simulink model "Project"  (R2020b)
settings: Solver=VariableStepAuto  StartTime=0.0  StopTime=100  RelTol=1e-3
undefined symbols (not defined in the file or in its folder): RES, SET, sigbuilder_block
settings Model: EnablePacing=on  PacingRate=2  Creator=99003729  LastModifiedBy=Admin

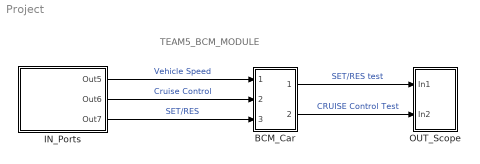
== system Project ==
  note: TEAM5_BCM_MODULE
  BCM_Car : Subsystem
  IN_Ports : Subsystem
  OUT_Scope : Subsystem
  wires:
  IN_Ports/1(Out5) -> BCM_Car/1(In1)  "Vehicle Speed"
  IN_Ports/3(Out7) -> BCM_Car/3(In3)  "SET/RES"
  IN_Ports/2(Out6) -> BCM_Car/2(In2)  "Cruise Control"
  BCM_Car/1(Out1) -> OUT_Scope/1(In1)  "SET/RES test"
  BCM_Car/2(Out2) -> OUT_Scope/2(In2)  "CRUISE Control Test"

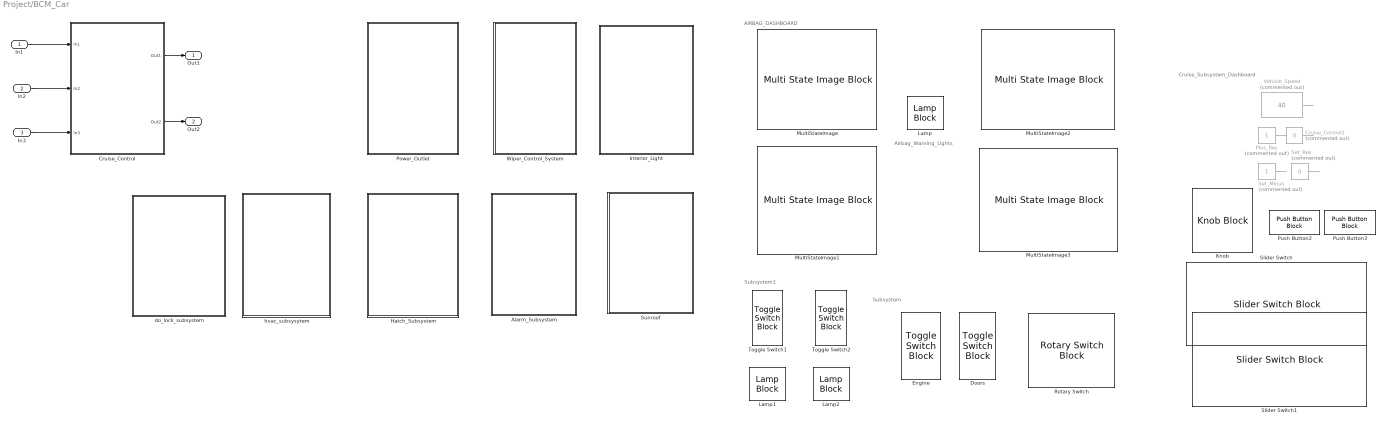
== system Project/BCM_Car ==
  note: AIRBAG_DASHBOARD
  note: Airbag_Warning_Lights
  note: Cruise_Subsystem_Dashboard
  note: Subsystem
  note: Subsystem1
  In1 : Inport
  In2 : Inport  Port=2
  In3 : Inport  Port=3
  Alarm_Subsystem : Subsystem
  Cruise_Control : Subsystem
  Cruise_Control1 : Constant  Commented=on  Value=0
  Doors : ToggleSwitchBlock
      settings: Values={{'Off', 'On'}, [0 1]}
  Engine : ToggleSwitchBlock
      settings: Values={{'Off', 'On'}, [0 1]}
  Hatch_Subsystem : Subsystem
  Interior_Light : Subsystem
  Knob : KnobBlock
  Lamp : LampBlock
  Lamp1 : LampBlock
  Lamp2 : LampBlock
  MultiStateImage{,1..3} (4 alike) : MultiStateImageBlock
  Plus_Res : Constant  Commented=on
  Power_Outlet : Subsystem
  Push Button2 : PushButtonBlock  ButtonText=SET-
  Push Button3 : PushButtonBlock  ButtonText=+RES
  Rotary Switch : RotarySwitchBlock
      settings: Values={{'Off', 'Button', 'Double Press'}, [0 1 2]}
  Set_Minus : Constant  Commented=on
  Set_Res : Constant  Commented=on  Value=0
  Slider Switch : SliderSwitchBlock
      settings: Values={{'Cruise Control Off', 'Cruise Control On'}, [0 1]}
  Slider Switch1 : SliderSwitchBlock
      settings: Values={{'Off with set speed', 'Resume set speed'}, [0 1]}
  Sunroof : Subsystem
  Toggle Switch1 : ToggleSwitchBlock
      settings: Values={{'Bonnet Off', 'Bonnet On'}, [0 1]}
  Toggle Switch2 : ToggleSwitchBlock
      settings: Values={{'Bonnet Off', 'Bonnet On'}, [0 1]}
  Vehicle_Speed : Constant  Commented=on  Value=40
  Wiper_Control_System : Subsystem
  do_lock_subsystem : Subsystem
  hvac_subsysytem : Subsystem
  Out1 : Outport
  Out2 : Outport  Port=2
  wires:
  Set_Res/1 -> ?
  Plus_Res/1 -> ?
  Vehicle_Speed/1 -> ?
  Set_Minus/1 -> ?
  Cruise_Control1/1 -> ?
  In1/1 -> Cruise_Control/1(In1)
  In2/1 -> Cruise_Control/2(In2)
  In3/1 -> Cruise_Control/3(In3)
  Cruise_Control/1(Out1) -> Out1/1
  Cruise_Control/2(Out2) -> Out2/1

== system Project/IN_Ports ==
  note: Airbag_And_Cruise_InPorts
  Alarm_and_Hatch_InPorts : Subsystem
  Hvac_and_Door_InPorts : Subsystem
  Square_Signals : Subsystem  Tag=STV Subsys  LoadFcn=sigbuilder_block('load');  StartFcn=sigbuilder_block('start');  StopFcn=sigbuilder_block('stop');  ClipboardFcn=sigbuilder_block('clipboard');  mask(Sigbuilder block){tuvar=[0:10]}
      mask help: Simulink:masks:SigbuilderBlock_MD
      mask init:
      | if ~strcmp(get_param(bdroot(gcbh),'SimulationStatus'),'stopped') tuvar = sigbuilder_block('maskInit'); end
      settings: CopyFcn=sigbuilder_block('copy');  DeleteFcn=sigbuilder_block('delete');  ModelCloseFcn=sigbuilder_block('modelClose');  PreSaveFcn=sigbuilder_block('preSave');  PauseFcn=sigbuilder_block('pause');  ContinueFcn=sigbuilder_block('continue');  NameChangeFcn=sigbuilder_block('namechange');  OpenFcn=sigbuilder_block('open',[6 30 1012.5 447.75 ]);  CloseFcn=sigbuilder_block('close');
      mask Display: plot(0, 0, 100, 100,[2, 2, 32, 32, 2], [68, 8, 8, 68, 68],[32, 2], [38, 38], [32, 19, 2],[53, 60, 44], [32, 17, 17, 2],[16, 16, 31, 31]);txt = getActiveGroup(gcbh);text(2, 100, txt,'verticalAlignment', 'top');
  Sunroof_and_InteriorLights_InPorts : Subsystem
  Wiper_and_Power_InPorts : Subsystem
  Out5 : Outport
  Out6 : Outport  Port=2
  Out7 : Outport  Port=3
  wires:
  Square_Signals/2(Cruise_Control) -> Out6/1  "Cruise_Control"
  Square_Signals/1(Vehicle_Speed) -> Out5/1  "Vehicle_Spped"
  Square_Signals/3(Set_Res_Control) -> Out7/1  "Set_Res_Control"

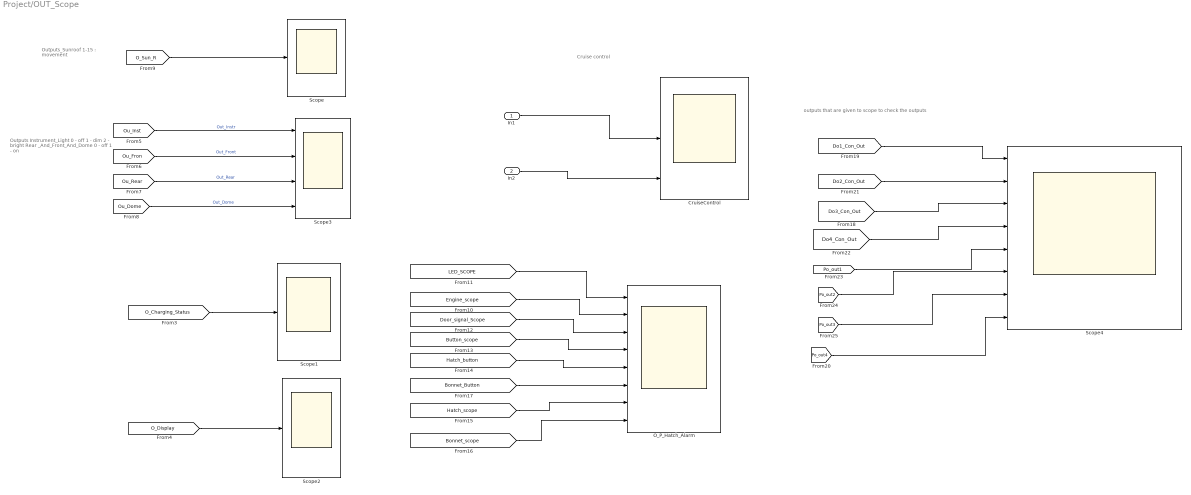
== system Project/OUT_Scope ==
  note: Cruise control
  note: Outputs
      | Instrument_Light
      | 0 - off
      | 1 - dim
      | 2 - bright
      | Rear _And_Front_And_Dome
      | 0 - off
      | 1 - on
  note: Outputs_Sunroof
      | 1-15 : movement
  note: outputs that are given to scope to check the outputs
  In1 : Inport
  In2 : Inport  Port=2
  CruiseControl : Scope  NumInputPorts=3
  O_P_Hatch_Alarm : Scope  NumInputPorts=8
  Scope : Scope
  Scope1 : Scope
  Scope2 : Scope
  Scope3 : Scope  NumInputPorts=4
  Scope4 : Scope  NumInputPorts=8
  wires:
  [O_Charging_Status] -> Scope1/1
  [O_Display] -> Scope2/1
  [Ou_Inst] -> Scope3/1  "Out_Instr"
  [Ou_Fron] -> Scope3/2  "Out_Front"
  [Ou_Rear] -> Scope3/3  "Out_Rear"
  [Ou_Dome] -> Scope3/4  "Out_Dome"
  [O_Sun_R] -> Scope/1
  [Bonnet_Button] -> O_P_Hatch_Alarm/6
  [Bonnet_scope] -> O_P_Hatch_Alarm/8
  [Door_signal_Scope] -> O_P_Hatch_Alarm/3
  [Hatch_button] -> O_P_Hatch_Alarm/5
  [Hatch_scope] -> O_P_Hatch_Alarm/7
  [LED_SCOPE] -> O_P_Hatch_Alarm/1
  [Engine_scope] -> O_P_Hatch_Alarm/2
  [Button_scope] -> O_P_Hatch_Alarm/4
  [Po_out3] -> Scope4/7
  [Po_out4] -> Scope4/8
  [Do3_Con_Out] -> Scope4/3
  [Po_out1] -> Scope4/5
  [Do1_Con_Out] -> Scope4/1
  [Do4_Con_Out] -> Scope4/4
  [Po_out2] -> Scope4/6
  [Do2_Con_Out] -> Scope4/2
  In1/1 -> CruiseControl/2
  In2/1 -> CruiseControl/3

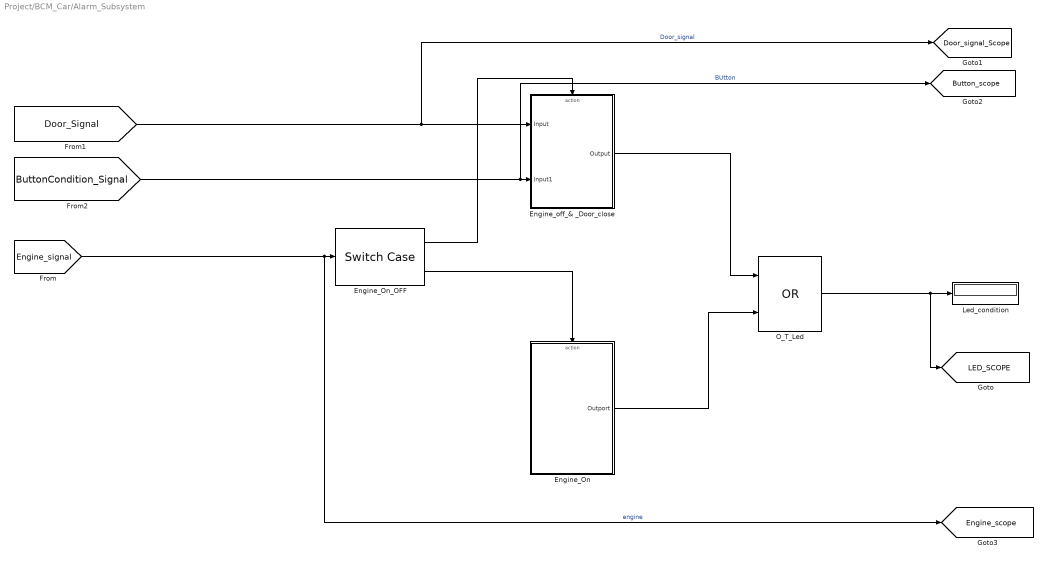
== system Project/BCM_Car/Alarm_Subsystem ==
  Engine_On : Subsystem  TreatAsAtomicUnit=on
  Engine_On_OFF : SwitchCase  CaseConditions={0,1}  ShowDefaultCase=off
  Engine_off_& _Door_close : Subsystem  TreatAsAtomicUnit=on
  Led_condition : Display
  O_T_Led : Logic  Operator=OR  IconShape=distinctive  AllPortsSameDT=off  OutDataTypeStr=boolean
  tag scope: Button_scope=global, Door_signal_Scope=global, Engine_scope=global, LED_SCOPE=global
  wires:
  O_T_Led/1 -> [LED_SCOPE], Led_condition/1
  Engine_On_OFF/1 -> Engine_off_& _Door_close/Action
  Engine_On_OFF/2 -> Engine_On/Action
  Engine_On/1(Outport) -> O_T_Led/2
  Engine_off_& _Door_close/1(Output) -> O_T_Led/1
  [Engine_signal] -> [Engine_scope], Engine_On_OFF/1  "engine"
  [Door_Signal] -> [Door_signal_Scope], Engine_off_& _Door_close/1(Input)  "Door_signal"
  [ButtonCondition_Signal] -> [Button_scope], Engine_off_& _Door_close/2(Input1)  "BUtton"

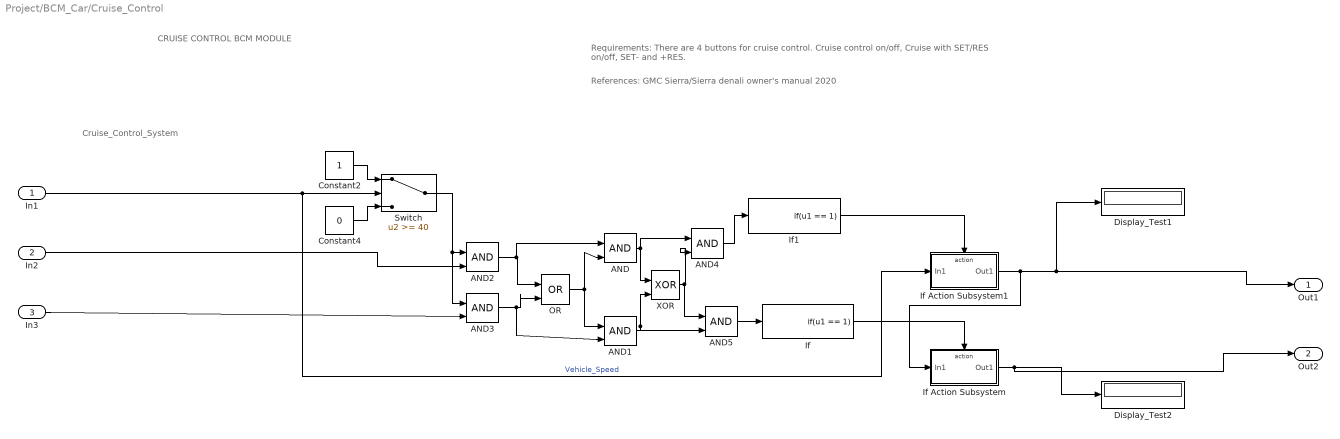
== system Project/BCM_Car/Cruise_Control ==
  note: Cruise_Control_System
  note: CRUISE CONTROL BCM MODULE
  note: References: GMC Sierra/Sierra denali owner's manual 2020
  note: Requirements: There are 4 buttons for cruise control. Cruise control on/off, Cruise with SET/RES on/off, SET- and +RES.
  In1 : Inport
  In2 : Inport  Port=2
  In3 : Inport  Port=3
  AND{,1..5} (6 alike) : Logic  IconShape=distinctive  AllPortsSameDT=off  OutDataTypeStr=boolean
  Constant2 : Constant
  Constant4 : Constant  Value=0
  Display_Test1 : Display
  Display_Test2 : Display
  If : If  IfExpression=u1 == 1  ShowElse=off
  If Action Subsystem : Subsystem  TreatAsAtomicUnit=on
  If Action Subsystem1 : Subsystem  TreatAsAtomicUnit=on
  If1 : If  IfExpression=u1 == 1  ShowElse=off
  OR : Logic  Operator=OR  IconShape=distinctive  AllPortsSameDT=off  OutDataTypeStr=boolean
  Switch : Switch  Threshold=40
  XOR : Logic  Operator=XOR  IconShape=distinctive  AllPortsSameDT=off  OutDataTypeStr=boolean
  Out1 : Outport
  Out2 : Outport  Port=2
  wires:
  In3/1 -> AND3/2
  AND5/1 -> If/1
  If1/1 -> If Action Subsystem1/Action
  If/1 -> If Action Subsystem/Action
  If Action Subsystem/1(Out1) -> Out2/1, Display_Test2/1
  AND/1 -> AND4/1, XOR/1
  XOR/1 -> AND5/1, AND4/2
  In1/1 -> If Action Subsystem1/1(In1), Switch/2  "Vehicle_Speed"
  OR/1 -> AND1/1, AND/2
  AND2/1 -> AND/1, OR/1
  In2/1 -> AND2/2
  Constant4/1 -> Switch/3
  AND3/1 -> AND1/2, OR/2
  AND1/1 -> XOR/2, AND5/2
  Switch/1 -> AND3/1, AND2/1
  Constant2/1 -> Switch/1
  AND4/1 -> If1/1
  If Action Subsystem1/1(Out1) -> If Action Subsystem/1(In1), Out1/1, Display_Test1/1

== system Project/BCM_Car/Hatch_Subsystem ==
  H_B_condition : Stateflow chart  TreatAsAtomicUnit=on
  Hatch_Bonnet_condition : Display
  OR : Logic  Operator=OR  IconShape=distinctive  AllPortsSameDT=off  OutDataTypeStr=boolean
  tag scope: Bonnet_scope=global, Hatch_scope=global
  wires:
  [Bonnet_Button] -> H_B_condition/1(BonnetButton)
  OR/1 -> Hatch_Bonnet_condition/1
  H_B_condition/1(y) -> [Bonnet_scope], OR/1
  H_B_condition/2(x) -> [Hatch_scope], OR/2
  [Hatch_button] -> H_B_condition/2(hatchButton)

== system Project/BCM_Car/Interior_Light ==
  Function_Light : MATLAB Function  TreatAsAtomicUnit=on
  tag scope: Ou_Dome=global, Ou_Fron=global, Ou_Inst=global, Ou_Rear=global
  wires:
  [Dome_L] -> Function_Light/4(u3)
  [Inst_Light] -> Function_Light/1(u)
  [Fron_Read_Light] -> Function_Light/2(u1)
  [Rear_Read_Light] -> Function_Light/3(u2)
  Function_Light/1(y) -> [Ou_Inst]
  Function_Light/2(y1) -> [Ou_Fron]
  Function_Light/3(y2) -> [Ou_Rear]
  Function_Light/4(y3) -> [Ou_Dome]

== system Project/BCM_Car/Power_Outlet ==
  note: Inputs_Engine
      |
      | 0: Engine is Off
      | 1: Engine is On
  I_Const_0 : Constant  Value=0
  I_Const_1 : Constant
  Power_Outlet_Subsystem : Subsystem
  Switch : Switch  Criteria=u2 > Threshold
  wires:
  I_Const_0/1 -> Switch/3
  [Engine_Input] -> Switch/2
  Switch/1 -> Power_Outlet_Subsystem/1(In1)
  I_Const_1/1 -> Switch/1

== system Project/BCM_Car/Sunroof ==
  Function_Sun : MATLAB Function  TreatAsAtomicUnit=on
  tag scope: O_Sun_R=global
  wires:
  Function_Sun/1(y) -> [O_Sun_R]  "Out_Sun"
  [I_Sensor] -> Function_Sun/2(v)
  [In_Su_Roof] -> Function_Sun/1(u)

== system Project/BCM_Car/Wiper_Control_System ==
  note: 1:Wiper is in Low Speed
      | 2:Wiper is in Medium Speed
      | 3:Wiper is in High Speed
      | 4:Wiper is in Mist
      | 5:Wiper is in OFF
  High_Speed : Constant  Value=3
  Low_Speed : Constant
  Medium_Speed : Constant  Value=2
  Mist : Constant  Value=4
  Multiport Switch for input conditions : MultiPortSwitch  Inputs=5  DiagnosticForDefault=None
  Off : Constant  Value=5
  tag scope: O_Display=global
  wires:
  [In_Value_Wiper] -> Multiport Switch for input conditions/1
  Low_Speed/1 -> Multiport Switch for input conditions/2
  Mist/1 -> Multiport Switch for input conditions/5
  Medium_Speed/1 -> Multiport Switch for input conditions/3
  Multiport Switch for input conditions/1 -> [O_Display]
  High_Speed/1 -> Multiport Switch for input conditions/4
  Off/1 -> Multiport Switch for input conditions/6

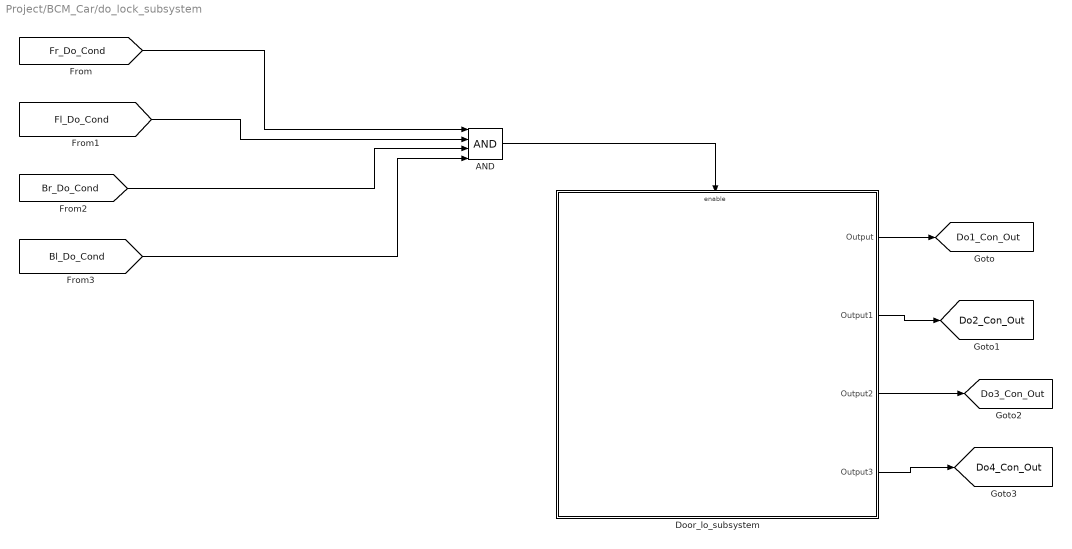
== system Project/BCM_Car/do_lock_subsystem ==
  AND : Logic  Inputs=4  IconShape=distinctive  AllPortsSameDT=off  OutDataTypeStr=boolean
  Door_lo_subsystem : Subsystem  TreatAsAtomicUnit=on
  tag scope: Do1_Con_Out=global, Do2_Con_Out=global, Do3_Con_Out=global, Do4_Con_Out=global
  wires:
  [Br_Do_Cond] -> AND/3
  [Fl_Do_Cond] -> AND/2
  [Fr_Do_Cond] -> AND/1
  AND/1 -> Door_lo_subsystem/Enable
  [Bl_Do_Cond] -> AND/4
  Door_lo_subsystem/1(Output) -> [Do1_Con_Out]
  Door_lo_subsystem/2(Output1) -> [Do2_Con_Out]
  Door_lo_subsystem/3(Output2) -> [Do3_Con_Out]
  Door_lo_subsystem/4(Output3) -> [Do4_Con_Out]

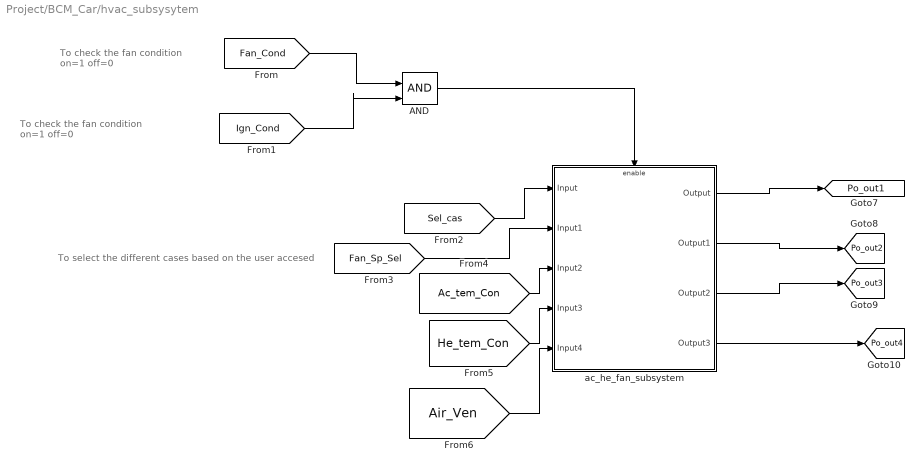
== system Project/BCM_Car/hvac_subsysytem ==
  note: To select the different cases based on the user accesed
  note: To check the fan condition
      | on=1
      | off=0
  note: To check the fan condition
      | on=1
      | off=0
  AND : Logic  IconShape=distinctive  AllPortsSameDT=off  OutDataTypeStr=boolean
  ac_he_fan_subsystem : Subsystem
  tag scope: Po_out1=global, Po_out2=global, Po_out3=global, Po_out4=global
  wires:
  [Fan_Cond] -> AND/1
  [Ign_Cond] -> AND/2
  AND/1 -> ac_he_fan_subsystem/Enable
  [Sel_cas] -> ac_he_fan_subsystem/1(Input)
  [Fan_Sp_Sel] -> ac_he_fan_subsystem/2(Input1)
  [Ac_tem_Con] -> ac_he_fan_subsystem/3(Input2)
  [He_tem_Con] -> ac_he_fan_subsystem/4(Input3)
  ac_he_fan_subsystem/1(Output) -> [Po_out1]
  ac_he_fan_subsystem/2(Output1) -> [Po_out2]
  ac_he_fan_subsystem/3(Output2) -> [Po_out3]
  ac_he_fan_subsystem/4(Output3) -> [Po_out4]
  [Air_Ven] -> ac_he_fan_subsystem/5(Input4)

== system Project/IN_Ports/Alarm_and_Hatch_InPorts ==
  Signal Builder : Subsystem  Tag=STV Subsys  LoadFcn=sigbuilder_block('load');  StartFcn=sigbuilder_block('start');  StopFcn=sigbuilder_block('stop');  ClipboardFcn=sigbuilder_block('clipboard');  mask(Sigbuilder block){tuvar=[0:10]}
      mask help: Simulink:masks:SigbuilderBlock_MD
      mask init:
      | if ~strcmp(get_param(bdroot(gcbh),'SimulationStatus'),'stopped') tuvar = sigbuilder_block('maskInit'); end
      settings: CopyFcn=sigbuilder_block('copy');  DeleteFcn=sigbuilder_block('delete');  ModelCloseFcn=sigbuilder_block('modelClose');  PreSaveFcn=sigbuilder_block('preSave');  PauseFcn=sigbuilder_block('pause');  ContinueFcn=sigbuilder_block('continue');  NameChangeFcn=sigbuilder_block('namechange');  OpenFcn=sigbuilder_block('open',[437.6 199.2 550.4 400 ]);  CloseFcn=sigbuilder_block('close');
      mask Display: plot(0, 0, 100, 100,[2, 2, 32, 32, 2], [68, 8, 8, 68, 68],[32, 2], [38, 38], [32, 19, 2],[53, 60, 44], [32, 17, 17, 2],[16, 16, 31, 31]);txt = getActiveGroup(gcbh);text(2, 100, txt,'verticalAlignment', 'top');
  tag scope: Bonnet_Button=global, ButtonCondition_Signal=global, Door_Signal=global, Engine_signal=global, Hatch_button=global
  wires:
  Signal Builder/1(Engine_Signal) -> [Engine_signal]
  Signal Builder/5(Hatch_button) -> [Hatch_button]
  Signal Builder/4(Bonnet_button) -> [Bonnet_Button]
  Signal Builder/2(Door_signal) -> [Door_Signal]
  Signal Builder/3(ButtonCondition_Signal) -> [ButtonCondition_Signal]

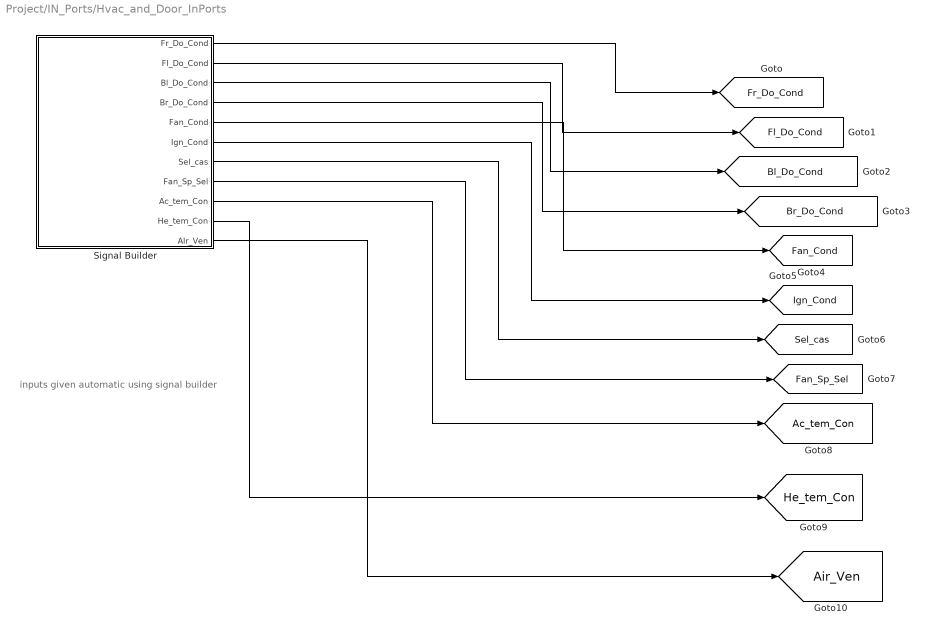
== system Project/IN_Ports/Hvac_and_Door_InPorts ==
  note: inputs given automatic using signal builder
  Signal Builder : Subsystem  Tag=STV Subsys  LoadFcn=sigbuilder_block('load');  StartFcn=sigbuilder_block('start');  StopFcn=sigbuilder_block('stop');  ClipboardFcn=sigbuilder_block('clipboard');  mask(Sigbuilder block){tuvar=[0:10]}
      mask help: Simulink:masks:SigbuilderBlock_MD
      mask init:
      | if ~strcmp(get_param(bdroot(gcbh),'SimulationStatus'),'stopped') tuvar = sigbuilder_block('maskInit'); end
      settings: CopyFcn=sigbuilder_block('copy');  DeleteFcn=sigbuilder_block('delete');  ModelCloseFcn=sigbuilder_block('modelClose');  PreSaveFcn=sigbuilder_block('preSave');  PauseFcn=sigbuilder_block('pause');  ContinueFcn=sigbuilder_block('continue');  NameChangeFcn=sigbuilder_block('namechange');  OpenFcn=sigbuilder_block('open',[544.5 115.5 550.5 399.75 ]);  CloseFcn=sigbuilder_block('close');
      mask Display: plot(0, 0, 100, 100,[2, 2, 32, 32, 2], [68, 8, 8, 68, 68],[32, 2], [38, 38], [32, 19, 2],[53, 60, 44], [32, 17, 17, 2],[16, 16, 31, 31]);txt = getActiveGroup(gcbh);text(2, 100, txt,'verticalAlignment', 'top');
  tag scope: Ac_tem_Con=global, Air_Ven=global, Bl_Do_Cond=global, Br_Do_Cond=global, Fan_Cond=global, Fan_Sp_Sel=global, Fl_Do_Cond=global, Fr_Do_Cond=global, He_tem_Con=global, Ign_Cond=global, Sel_cas=global
  wires:
  Signal Builder/4(Br_Do_Cond) -> [Br_Do_Cond]
  Signal Builder/2(Fl_Do_Cond) -> [Fl_Do_Cond]
  Signal Builder/6(Ign_Cond) -> [Ign_Cond]
  Signal Builder/3(Bl_Do_Cond) -> [Bl_Do_Cond]
  Signal Builder/7(Sel_cas) -> [Sel_cas]
  Signal Builder/8(Fan_Sp_Sel) -> [Fan_Sp_Sel]
  Signal Builder/1(Fr_Do_Cond) -> [Fr_Do_Cond]
  Signal Builder/5(Fan_Cond) -> [Fan_Cond]
  Signal Builder/9(Ac_tem_Con) -> [Ac_tem_Con]
  Signal Builder/11(AIr_Ven) -> [Air_Ven]
  Signal Builder/10(He_tem_Con) -> [He_tem_Con]

== system Project/IN_Ports/Square_Signals ==
  Demux : Demux  Tag=STV Demux  Outputs=3
      settings: DisplayOption=none
  FromWs : FromWorkspace  Tag=STV FromWs  VariableName=tuvar
      SigBuilderData=|
      | common.afterFinalStr = 'Extrapolate'
      | common.sampleTime = 0
      | dataSet.timeRange = [0 100]
      | dataSet.name = 'Group 1'
      | sbobj.Groups.Name = 'Group 1'
      | sbobj.Groups.Signals(1).Name = 'Vehicle_Speed'
      | sbobj.Groups.Signals(1).XData = [0 5 10 15 20 25 30 35 40 45 50 55 60 65 70 75 80 85 90 95 100]
      | sbobj.Groups.Signals(1).YData = [50 50 50 50 50 50 50 50 50 50 50 50 50 50 50 50 50 50 50 50 50]
      | sbobj.Groups.Signals(2).Name = 'Cruise_Control'
      | sbobj.Groups.Signals(2).XData = [0 5 5 10 15 20 25 30 35 40 45 50 55 60 65 70 75 80 85 90 95 100]
      | sbobj.Groups.Signals(2).YData = [0 0 1 1 1 1 1 0 0 0 0 0 0 0 0 0 0 0 0 0 0 0]
      | sbobj.Groups.Signals(3).Name = 'Set_Res_Control'
      | sbobj.Groups.Signals(3).XData = [0 5 10 15 20 25 30 30 35 35 40 45 50 55 60 65 70 75 80 85 90 95 100]
      | sbobj.Groups.Signals(3).YData = [0 0 0 0 0 0 0 1 1 0 0 0 0 0 0 0 0 0 0 0 0 0 0]
      | sbobj.Groups.TimeRange = [0 100]
  Vehicle_Speed : Outport  Tag=STV Outport
  Cruise_Control : Outport  Tag=STV Outport  Port=2
  Set_Res_Control : Outport  Tag=STV Outport  Port=3
  wires:
  FromWs/1 -> Demux/1
  Demux/1 -> Vehicle_Speed/1
  Demux/2 -> Cruise_Control/1
  Demux/3 -> Set_Res_Control/1

== system Project/IN_Ports/Sunroof_and_InteriorLights_InPorts ==
  note: Inputs
      | Intrument_Light
      | 0 - off
      | 1 - dim
      | 2- bright
      | Front_And_Rear_Light
      | 0 - off
      | 1 - on
      | Dome_Light
      | 0 - off
      | 1 - on
  note: Sunroof_Inputs
      | 0 - off
      | 1 - siglepress
      | 2 - fullpress
      | Sensor_For_Object
      | 0 - no object
      | 1 - object
  Signal Builder2 : Subsystem  Tag=STV Subsys  LoadFcn=sigbuilder_block('load');  StartFcn=sigbuilder_block('start');  StopFcn=sigbuilder_block('stop');  ClipboardFcn=sigbuilder_block('clipboard');  mask(Sigbuilder block){tuvar=[0:10]}
      mask help: Simulink:masks:SigbuilderBlock_MD
      mask init:
      | if ~strcmp(get_param(bdroot(gcbh),'SimulationStatus'),'stopped') tuvar = sigbuilder_block('maskInit'); end
      settings: CopyFcn=sigbuilder_block('copy');  DeleteFcn=sigbuilder_block('delete');  ModelCloseFcn=sigbuilder_block('modelClose');  PreSaveFcn=sigbuilder_block('preSave');  PauseFcn=sigbuilder_block('pause');  ContinueFcn=sigbuilder_block('continue');  NameChangeFcn=sigbuilder_block('namechange');  OpenFcn=sigbuilder_block('open',[373.5 207 544.5 355.5 ]);  CloseFcn=sigbuilder_block('close');
      mask Display: plot(0, 0, 100, 100,[2, 2, 32, 32, 2], [68, 8, 8, 68, 68],[32, 2], [38, 38], [32, 19, 2],[53, 60, 44], [32, 17, 17, 2],[16, 16, 31, 31]);txt = getActiveGroup(gcbh);text(2, 100, txt,'verticalAlignment', 'top');
  Signal Builder3 : Subsystem  Tag=STV Subsys  LoadFcn=sigbuilder_block('load');  StartFcn=sigbuilder_block('start');  StopFcn=sigbuilder_block('stop');  ClipboardFcn=sigbuilder_block('clipboard');  mask(Sigbuilder block){tuvar=[0:10]}
      mask help: Simulink:masks:SigbuilderBlock_MD
      mask init:
      | if ~strcmp(get_param(bdroot(gcbh),'SimulationStatus'),'stopped') tuvar = sigbuilder_block('maskInit'); end
      settings: CopyFcn=sigbuilder_block('copy');  DeleteFcn=sigbuilder_block('delete');  ModelCloseFcn=sigbuilder_block('modelClose');  PreSaveFcn=sigbuilder_block('preSave');  PauseFcn=sigbuilder_block('pause');  ContinueFcn=sigbuilder_block('continue');  NameChangeFcn=sigbuilder_block('namechange');  OpenFcn=sigbuilder_block('open',[591 352.5 550.5 359.25 ]);  CloseFcn=sigbuilder_block('close');
      mask Display: plot(0, 0, 100, 100,[2, 2, 32, 32, 2], [68, 8, 8, 68, 68],[32, 2], [38, 38], [32, 19, 2],[53, 60, 44], [32, 17, 17, 2],[16, 16, 31, 31]);txt = getActiveGroup(gcbh);text(2, 100, txt,'verticalAlignment', 'top');
  tag scope: Dome_L=global, Fron_Read_Light=global, I_Sensor=global, In_Su_Roof=global, Inst_Light=global, Rear_Read_Light=global
  wires:
  Signal Builder2/1(Fron_Read_Light) -> [Fron_Read_Light]
  Signal Builder3/2(I_Sensor) -> [I_Sensor]
  Signal Builder2/3(Dome_L) -> [Dome_L]
  Signal Builder2/2(Rear_Read_Light) -> [Rear_Read_Light]
  Signal Builder3/1(In_Su_Roof) -> [In_Su_Roof]
  Signal Builder2/4(Inst_Light) -> [Inst_Light]

== system Project/IN_Ports/Wiper_and_Power_InPorts ==
  note: Inputs_Engine
      |
      | 0: Engine is Off
      | 1: Engine is On
  note: Input_Wiper_Control
      | 1:Low Speed
      | 2:Medium Speed
      | 3:High Speed
      | 4:Mist
      | 5:Off
  Signal Builder : Subsystem  Tag=STV Subsys  LoadFcn=sigbuilder_block('load');  StartFcn=sigbuilder_block('start');  StopFcn=sigbuilder_block('stop');  ClipboardFcn=sigbuilder_block('clipboard');  mask(Sigbuilder block){tuvar=[0:10]}
      mask help: Simulink:masks:SigbuilderBlock_MD
      mask init:
      | if ~strcmp(get_param(bdroot(gcbh),'SimulationStatus'),'stopped') tuvar = sigbuilder_block('maskInit'); end
      settings: CopyFcn=sigbuilder_block('copy');  DeleteFcn=sigbuilder_block('delete');  ModelCloseFcn=sigbuilder_block('modelClose');  PreSaveFcn=sigbuilder_block('preSave');  PauseFcn=sigbuilder_block('pause');  ContinueFcn=sigbuilder_block('continue');  NameChangeFcn=sigbuilder_block('namechange');  OpenFcn=sigbuilder_block('open',[197.25 223.5 550.5 359.25 ]);  CloseFcn=sigbuilder_block('close');
      mask Display: plot(0, 0, 100, 100,[2, 2, 32, 32, 2], [68, 8, 8, 68, 68],[32, 2], [38, 38], [32, 19, 2],[53, 60, 44], [32, 17, 17, 2],[16, 16, 31, 31]);txt = getActiveGroup(gcbh);text(2, 100, txt,'verticalAlignment', 'top');
  Signal Builder1 : Subsystem  Tag=STV Subsys  LoadFcn=sigbuilder_block('load');  StartFcn=sigbuilder_block('start');  StopFcn=sigbuilder_block('stop');  ClipboardFcn=sigbuilder_block('clipboard');  mask(Sigbuilder block){tuvar=[0:10]}
      mask help: Simulink:masks:SigbuilderBlock_MD
      mask init:
      | if ~strcmp(get_param(bdroot(gcbh),'SimulationStatus'),'stopped') tuvar = sigbuilder_block('maskInit'); end
      settings: CopyFcn=sigbuilder_block('copy');  DeleteFcn=sigbuilder_block('delete');  ModelCloseFcn=sigbuilder_block('modelClose');  PreSaveFcn=sigbuilder_block('preSave');  PauseFcn=sigbuilder_block('pause');  ContinueFcn=sigbuilder_block('continue');  NameChangeFcn=sigbuilder_block('namechange');  OpenFcn=sigbuilder_block('open',[0.75 30.75 718.5 715.5 ]);  CloseFcn=sigbuilder_block('close');
      mask Display: plot(0, 0, 100, 100,[2, 2, 32, 32, 2], [68, 8, 8, 68, 68],[32, 2], [38, 38], [32, 19, 2],[53, 60, 44], [32, 17, 17, 2],[16, 16, 31, 31]);txt = getActiveGroup(gcbh);text(2, 100, txt,'verticalAlignment', 'top');
  tag scope: Engine_Input=global, In_Value_Wiper=global
  wires:
  Signal Builder1/1(In_Value_Wiper) -> [In_Value_Wiper]
  Signal Builder/1(Engine_Input) -> [Engine_Input]

== system Project/BCM_Car/Alarm_Subsystem/Engine_On ==
  Action Port : ActionPort  ActionPortLabel=case [ 1 ]:
  Enigine_Off : Constant  Value=0
  Outport : Outport
  wires:
  Enigine_Off/1 -> Outport/1

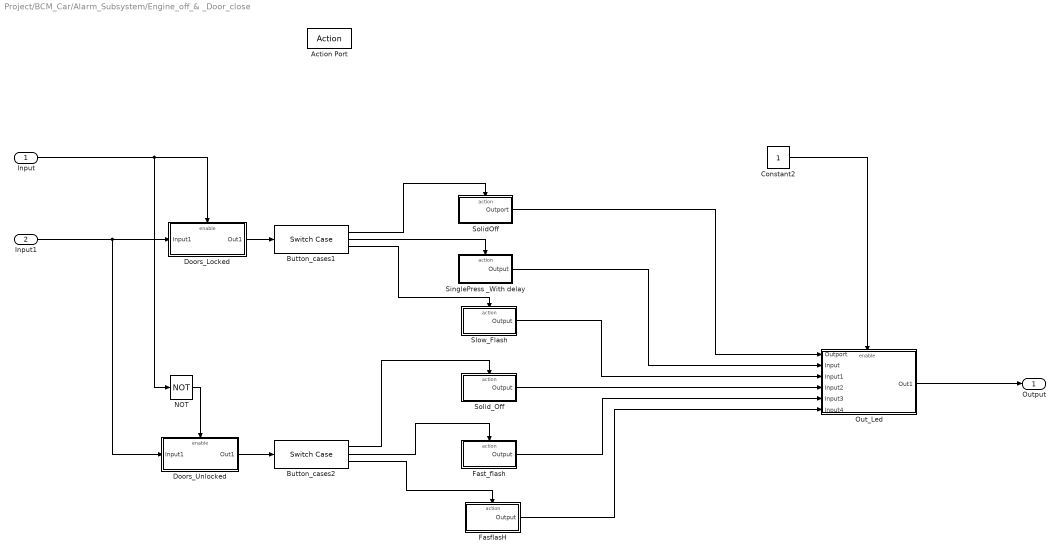
== system Project/BCM_Car/Alarm_Subsystem/Engine_off_& _Door_close ==
  Input : Inport
  Input1 : Inport  Port=2
  Action Port : ActionPort  ActionPortLabel=case [ 0 ]:
  " SolidOff" : Subsystem  TreatAsAtomicUnit=on
  Button_cases1 : SwitchCase  CaseConditions={0,1,2}  ShowDefaultCase=off
  Button_cases2 : SwitchCase  CaseConditions={0,1,2}  ShowDefaultCase=off
  Constant2 : Constant
  Doors_Locked : Subsystem  TreatAsAtomicUnit=on
  Doors_Unlocked : Subsystem  TreatAsAtomicUnit=on
  FasflasH : Subsystem  TreatAsAtomicUnit=on
  Fast_flash : Subsystem  TreatAsAtomicUnit=on
  NOT : Logic  Operator=NOT  IconShape=distinctive  AllPortsSameDT=off  OutDataTypeStr=boolean
  Out_Led : Subsystem  TreatAsAtomicUnit=on
  SinglePress _With delay : Subsystem  TreatAsAtomicUnit=on
  Slow_Flash : Subsystem  TreatAsAtomicUnit=on
  Solid_Off : Subsystem  TreatAsAtomicUnit=on
  Output : Outport
  wires:
  Out_Led/1(Out1) -> Output/1
  Button_cases1/1 -> " SolidOff"/Action
  Button_cases1/2 -> SinglePress _With delay/Action
  Button_cases1/3 -> Slow_Flash/Action
  Doors_Locked/1(Out1) -> Button_cases1/1
  NOT/1 -> Doors_Unlocked/Enable
  Doors_Unlocked/1(Out1) -> Button_cases2/1
  Button_cases2/1 -> Solid_Off/Action
  Button_cases2/2 -> Fast_flash/Action
  Button_cases2/3 -> FasflasH/Action
  Constant2/1 -> Out_Led/Enable
  Slow_Flash/1(Output) -> Out_Led/3(Input1)
  Fast_flash/1(Output) -> Out_Led/5(Input3)
  FasflasH/1(Output) -> Out_Led/6(Input4)
  SinglePress _With delay/1(Output) -> Out_Led/2(Input)
  Solid_Off/1(Output) -> Out_Led/4(Input2)
  " SolidOff"/1(Outport) -> Out_Led/1(Outport)
  Input/1 -> NOT/1, Doors_Locked/Enable
  Input1/1 -> Doors_Unlocked/1(Input1), Doors_Locked/1(Input1)

== system Project/BCM_Car/Cruise_Control/If Action Subsystem ==
  In1 : Inport
  Action Port : ActionPort  ActionPortLabel=if(u1 == 1)
  Out1 : Outport
  wires:
  In1/1 -> Out1/1

== system Project/BCM_Car/Cruise_Control/If Action Subsystem1 ==
  In1 : Inport
  Action Port : ActionPort  ActionPortLabel=if(u1 == 1)
  Add : Sum
  Chart : Stateflow chart  TreatAsAtomicUnit=on
  Signal Builder : Subsystem  Tag=STV Subsys  LoadFcn=sigbuilder_block('load');  StartFcn=sigbuilder_block('start');  StopFcn=sigbuilder_block('stop');  ClipboardFcn=sigbuilder_block('clipboard');  mask(Sigbuilder block){tuvar=[0:10]}
      mask help: Simulink:masks:SigbuilderBlock_MD
      mask init:
      | if ~strcmp(get_param(bdroot(gcbh),'SimulationStatus'),'stopped') tuvar = sigbuilder_block('maskInit'); end
      settings: CopyFcn=sigbuilder_block('copy');  DeleteFcn=sigbuilder_block('delete');  ModelCloseFcn=sigbuilder_block('modelClose');  PreSaveFcn=sigbuilder_block('preSave');  PauseFcn=sigbuilder_block('pause');  ContinueFcn=sigbuilder_block('continue');  NameChangeFcn=sigbuilder_block('namechange');  OpenFcn=sigbuilder_block('open',[0.75 30.75 718.5 715.5 ]);  CloseFcn=sigbuilder_block('close');
      mask Display: plot(0, 0, 100, 100,[2, 2, 32, 32, 2], [68, 8, 8, 68, 68],[32, 2], [38, 38], [32, 19, 2],[53, 60, 44], [32, 17, 17, 2],[16, 16, 31, 31]);txt = getActiveGroup(gcbh);text(2, 100, txt,'verticalAlignment', 'top');
  Out1 : Outport
  wires:
  Signal Builder/1(Plus_Or_Resume) -> Chart/2(inc)
  Add/1 -> Out1/1
  Signal Builder/2(Set_Or_Minus) -> Chart/1(dec)
  Chart/1(data) -> Add/1
  In1/1 -> Add/2

== system Project/BCM_Car/Power_Outlet/Power_Outlet_Subsystem ==
  note: If engine is ON and Charging port is ON, then device starts charging
  In1 : Inport
  AND condition(if both are high) : Logic  IconShape=distinctive  AllPortsSameDT=off  OutDataTypeStr=boolean
  Charging_Port : Constant
  Charging_Subsystem : Subsystem
  wires:
  In1/1 -> AND condition(if both are high)/1
  Charging_Port/1 -> AND condition(if both are high)/2
  AND condition(if both are high)/1 -> Charging_Subsystem/1(In1)

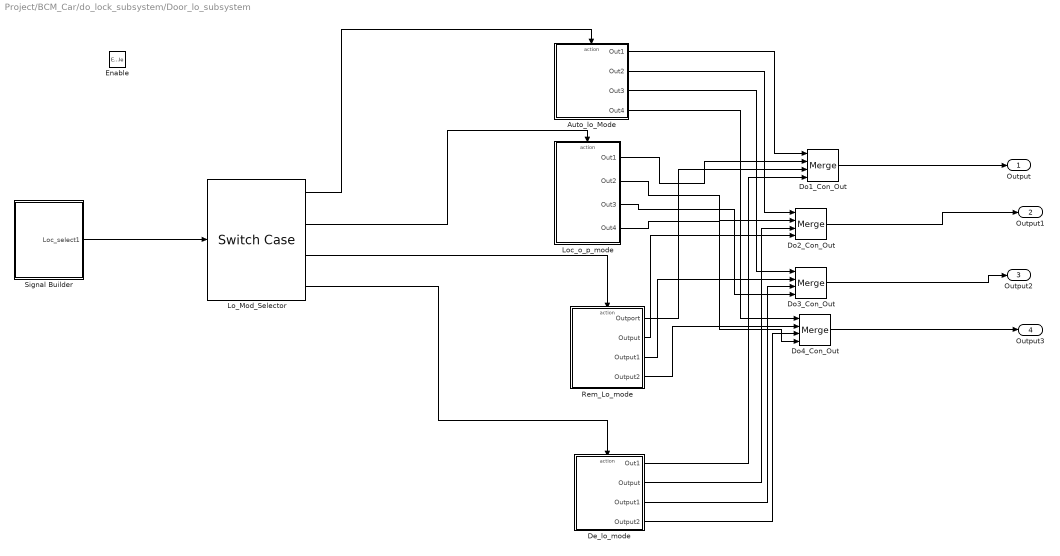
== system Project/BCM_Car/do_lock_subsystem/Door_lo_subsystem ==
  Enable : EnablePort
  Auto_lo_Mode : Subsystem  TreatAsAtomicUnit=on
  De_lo_mode : Subsystem  TreatAsAtomicUnit=on
  Do1_Con_Out : Merge  Inputs=4
  Do2_Con_Out : Merge  Inputs=4
  Do3_Con_Out : Merge  Inputs=4
  Do4_Con_Out : Merge  Inputs=4
  Lo_Mod_Selector : SwitchCase  CaseConditions={1,2,3,4}  ShowDefaultCase=off
  Loc_o_p_mode : Subsystem  TreatAsAtomicUnit=on
  Rem_Lo_mode : Subsystem  TreatAsAtomicUnit=on
  Signal Builder : Subsystem  Tag=STV Subsys  LoadFcn=sigbuilder_block('load');  StartFcn=sigbuilder_block('start');  StopFcn=sigbuilder_block('stop');  ClipboardFcn=sigbuilder_block('clipboard');  mask(Sigbuilder block){tuvar=[0:10]}
      mask help: Simulink:masks:SigbuilderBlock_MD
      mask init:
      | if ~strcmp(get_param(bdroot(gcbh),'SimulationStatus'),'stopped') tuvar = sigbuilder_block('maskInit'); end
      settings: CopyFcn=sigbuilder_block('copy');  DeleteFcn=sigbuilder_block('delete');  ModelCloseFcn=sigbuilder_block('modelClose');  PreSaveFcn=sigbuilder_block('preSave');  PauseFcn=sigbuilder_block('pause');  ContinueFcn=sigbuilder_block('continue');  NameChangeFcn=sigbuilder_block('namechange');  OpenFcn=sigbuilder_block('open',[437.6 199.2 550.4 400 ]);  CloseFcn=sigbuilder_block('close');
      mask Display: plot(0, 0, 100, 100,[2, 2, 32, 32, 2], [68, 8, 8, 68, 68],[32, 2], [38, 38], [32, 19, 2],[53, 60, 44], [32, 17, 17, 2],[16, 16, 31, 31]);txt = getActiveGroup(gcbh);text(2, 100, txt,'verticalAlignment', 'top');
  Output : Outport
  Output1 : Outport  Port=2
  Output2 : Outport  Port=3
  Output3 : Outport  Port=4
  wires:
  Signal Builder/1(Loc_select1) -> Lo_Mod_Selector/1
  Lo_Mod_Selector/3 -> Rem_Lo_mode/Action
  Lo_Mod_Selector/2 -> Loc_o_p_mode/Action
  Lo_Mod_Selector/1 -> Auto_lo_Mode/Action
  Auto_lo_Mode/1(Out1) -> Do1_Con_Out/1
  Loc_o_p_mode/1(Out1) -> Do1_Con_Out/2
  Auto_lo_Mode/2(Out2) -> Do2_Con_Out/1
  Loc_o_p_mode/2(Out2) -> Do2_Con_Out/2
  Auto_lo_Mode/3(Out3) -> Do3_Con_Out/1
  Loc_o_p_mode/3(Out3) -> Do3_Con_Out/4
  Auto_lo_Mode/4(Out4) -> Do4_Con_Out/1
  Loc_o_p_mode/4(Out4) -> Do4_Con_Out/4
  Rem_Lo_mode/1(Outport) -> Do1_Con_Out/3
  Rem_Lo_mode/2(Output) -> Do2_Con_Out/4
  Rem_Lo_mode/3(Output1) -> Do3_Con_Out/2
  Rem_Lo_mode/4(Output2) -> Do4_Con_Out/2
  Do1_Con_Out/1 -> Output/1
  Do2_Con_Out/1 -> Output1/1
  Do3_Con_Out/1 -> Output2/1
  Do4_Con_Out/1 -> Output3/1
  Lo_Mod_Selector/4 -> De_lo_mode/Action
  De_lo_mode/1(Out1) -> Do1_Con_Out/4
  De_lo_mode/2(Output) -> Do2_Con_Out/3
  De_lo_mode/3(Output1) -> Do3_Con_Out/3
  De_lo_mode/4(Output2) -> Do4_Con_Out/3

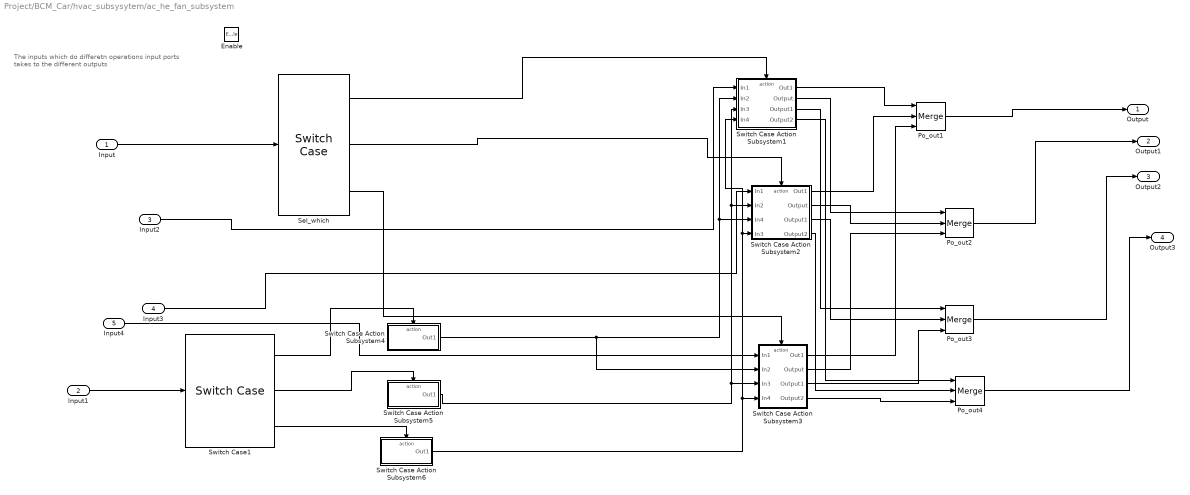
== system Project/BCM_Car/hvac_subsysytem/ac_he_fan_subsystem ==
  note: The inputs which do differetn operations
      | input ports takes to the different outputs
  Input : Inport
  Input1 : Inport  Port=2
  Input2 : Inport  Port=3
  Input3 : Inport  Port=4
  Input4 : Inport  Port=5
  Enable : EnablePort
  Po_out{1..4} (4 alike) : Merge  Inputs=3
  "Sel_which " : SwitchCase  CaseConditions={1,2,3}  ShowDefaultCase=off
  Switch Case Action Subsystem1 : Subsystem  TreatAsAtomicUnit=on
  Switch Case Action Subsystem2 : Subsystem  TreatAsAtomicUnit=on
  Switch Case Action Subsystem3 : Subsystem  TreatAsAtomicUnit=on
  Switch Case Action Subsystem4 : Subsystem  TreatAsAtomicUnit=on
  Switch Case Action Subsystem5 : Subsystem  TreatAsAtomicUnit=on
  Switch Case Action Subsystem6 : Subsystem  TreatAsAtomicUnit=on
  Switch Case1 : SwitchCase  CaseConditions={1,2,3}  ShowDefaultCase=off
  Output : Outport
  Output1 : Outport  Port=2
  Output2 : Outport  Port=3
  Output3 : Outport  Port=4
  wires:
  Input/1 -> "Sel_which "/1
  Input2/1 -> Switch Case Action Subsystem1/1(In1)
  Input3/1 -> Switch Case Action Subsystem2/1(In1)
  Input4/1 -> Switch Case Action Subsystem3/1(In1)
  Input1/1 -> Switch Case1/1
  Switch Case1/2 -> Switch Case Action Subsystem5/Action
  Switch Case1/1 -> Switch Case Action Subsystem4/Action
  Switch Case1/3 -> Switch Case Action Subsystem6/Action
  Switch Case Action Subsystem4/1(Out1) -> Switch Case Action Subsystem3/2(In2), Switch Case Action Subsystem1/2(In2), Switch Case Action Subsystem2/3(In4)
  Switch Case Action Subsystem5/1(Out1) -> Switch Case Action Subsystem1/3(In3), Switch Case Action Subsystem2/2(In2), Switch Case Action Subsystem3/3(In3)
  Switch Case Action Subsystem6/1(Out1) -> Switch Case Action Subsystem3/4(In4), Switch Case Action Subsystem1/4(In4), Switch Case Action Subsystem2/4(In3)
  "Sel_which "/1 -> Switch Case Action Subsystem1/Action
  "Sel_which "/2 -> Switch Case Action Subsystem2/Action
  "Sel_which "/3 -> Switch Case Action Subsystem3/Action
  Switch Case Action Subsystem1/1(Out1) -> Po_out1/1
  Switch Case Action Subsystem2/1(Out1) -> Po_out1/2
  Switch Case Action Subsystem3/1(Out1) -> Po_out1/3
  Switch Case Action Subsystem1/2(Output) -> Po_out2/1
  Switch Case Action Subsystem2/2(Output) -> Po_out2/2
  Switch Case Action Subsystem3/2(Output) -> Po_out2/3
  Switch Case Action Subsystem1/3(Output1) -> Po_out3/1
  Switch Case Action Subsystem2/3(Output1) -> Po_out3/2
  Switch Case Action Subsystem3/3(Output1) -> Po_out3/3
  Switch Case Action Subsystem1/4(Output2) -> Po_out4/1
  Switch Case Action Subsystem2/4(Output2) -> Po_out4/2
  Switch Case Action Subsystem3/4(Output2) -> Po_out4/3
  Po_out1/1 -> Output/1
  Po_out2/1 -> Output1/1
  Po_out3/1 -> Output2/1
  Po_out4/1 -> Output3/1

== system Project/IN_Ports/Alarm_and_Hatch_InPorts/Signal Builder ==
  Demux : Demux  Tag=STV Demux  Outputs=5
      settings: DisplayOption=none
  FromWs : FromWorkspace  Tag=STV FromWs  VariableName=tuvar
      SigBuilderData=|
      | common.afterFinalStr = 'Extrapolate'
      | common.sampleTime = 0
      | dataSet.timeRange = [0 10]
      | dataSet.name = 'Group 1'
      | sbobj.Groups.Name = 'Group 1'
      | sbobj.Groups.Signals(1).Name = 'Engine_Signal'
      | sbobj.Groups.Signals(1).XData = [0 5 5 10 10 15 15 20 20 25 25 30 30 35 35 40 40 45 45 50 50 55 55 60 60 65 65 70 70 75 75 80 80 85 85 90 90 95 95 100]
      | sbobj.Groups.Signals(1).YData = [0 0 1 1 0 0 1 1 0 0 1 1 0 0 1 1 0 0 1 1 0 0 1 1 0 0 1 1 0 0 1 1 0 0 1 1 0 0 1 1]
      | sbobj.Groups.Signals(2).Name = 'Door_signal'
      | sbobj.Groups.Signals(2).XData = [0 5 5 10 10 15 15 20 20 25 25 30 30 35 35 40 40 45 45 50 50 55 55 60 60 65 65 70 70 75 75 80 80 85 85 90 90 95 95 100]
      | sbobj.Groups.Signals(2).YData = [1 1 0 0 1 1 0 0 1 1 0 0 1 1 0 0 1 1 0 0 1 1 0 0 1 1 0 0 1 1 0 0 1 1 0 0 1 1 0 0]
      | sbobj.Groups.Signals(3).Name = 'ButtonCondition_Signal'
      | sbobj.Groups.Signals(3).XData = [0 5 5 10 15 20 20 25 30 35 35 40 40 45 45 50 50 55 60 60 65 65 70 70 75 75 80 85 90 95 95 100]
      | sbobj.Groups.Signals(3).YData = [0 0 1 2 2 0 1 2 2 0 1 2 0 1 2 0 1 1 1 2 0 1 2 0 1 2 1 1 1 0 1 1]
      | sbobj.Groups.Signals(4).Name = 'Bonnet_button'
      | sbobj.Groups.Signals(4).XData = [0 5 5 10 10 15 15 20 20 25 25 30 30 35 35 40 40 45 45 50 50 55 55 60 60 65 65 70 70 75 75 80 80 85 85 90 90 95 95 100]
      | sbobj.Groups.Signals(4).YData = [0 0 1 1 0 0 1 1 0 0 1 1 0 0 1 1 0 0 1 1 0 0 1 1 0 0 1 1 0 0 1 1 0 0 1 1 0 0 1 1]
      | sbobj.Groups.Signals(5).Name = 'Hatch_button'
      | sbobj.Groups.Signals(5).XData = [0 5 5 10 10 15 15 20 20 25 25 30 30 35 35 40 40 45 45 50 50 55 55 60 60 65 65 70 70 75 75 80 80 85 85 90 90 95 95 100]
      | sbobj.Groups.Signals(5).YData = [1 1 0 0 1 1 0 0 1 1 0 0 1 1 0 0 1 1 0 0 1 1 0 0 1 1 0 0 1 1 0 0 1 1 0 0 1 1 0 0]
      | sbobj.Groups.TimeRange = [0 100]
  Engine_Signal : Outport  Tag=STV Outport
  Door_signal : Outport  Tag=STV Outport  Port=2
  ButtonCondition_Signal : Outport  Tag=STV Outport  Port=3
  Bonnet_button : Outport  Tag=STV Outport  Port=4
  Hatch_button : Outport  Tag=STV Outport  Port=5
  wires:
  FromWs/1 -> Demux/1
  Demux/1 -> Engine_Signal/1
  Demux/2 -> Door_signal/1
  Demux/3 -> ButtonCondition_Signal/1
  Demux/4 -> Bonnet_button/1
  Demux/5 -> Hatch_button/1

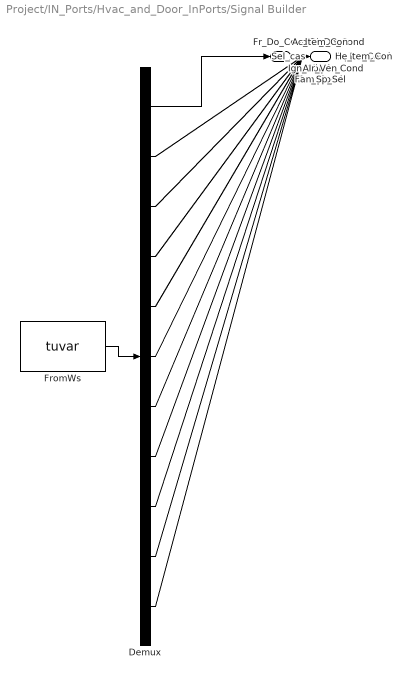
== system Project/IN_Ports/Hvac_and_Door_InPorts/Signal Builder ==
  Demux : Demux  Tag=STV Demux  Outputs=11
      settings: DisplayOption=none
  FromWs : FromWorkspace  Tag=STV FromWs  VariableName=tuvar
      SigBuilderData=|
      | common.afterFinalStr = 'Extrapolate'
      | common.sampleTime = 0
      | dataSet.timeRange = [0 10]
      | dataSet.name = 'Group 1'
      | sbobj.Groups.Name = 'Group 1'
      | sbobj.Groups.Signals(1).Name = 'Fr_Do_Cond'
      | sbobj.Groups.Signals(1).XData = [0 5 10 15 20 25 30 35 40]
      | sbobj.Groups.Signals(1).YData = [0 0 1 1 1 1 1 1 1]
      | sbobj.Groups.Signals(2).Name = 'Fl_Do_Cond'
      | sbobj.Groups.Signals(2).XData = [0 5 10 15 20 25 30 35 40]
      | sbobj.Groups.Signals(2).YData = [0 0 1 1 1 1 1 1 1]
      | sbobj.Groups.Signals(3).Name = 'Bl_Do_Cond'
      | sbobj.Groups.Signals(3).XData = [0 5 10 15 20 25 30 35 40]
      | sbobj.Groups.Signals(3).YData = [0 0 1 1 1 1 1 1 1]
      | sbobj.Groups.Signals(4).Name = 'Br_Do_Cond'
      | sbobj.Groups.Signals(4).XData = [0 5 10 15 20 25 30 35 40]
      | sbobj.Groups.Signals(4).YData = [0 0 1 1 1 1 1 1 1]
      | sbobj.Groups.Signals(5).Name = 'Fan_Cond'
      | sbobj.Groups.Signals(5).XData = [0 5 10 15 20 25 30 35 40]
      | sbobj.Groups.Signals(5).YData = [0 0 1 1 1 1 1 1 1]
      | sbobj.Groups.Signals(6).Name = 'Ign_Cond'
      | sbobj.Groups.Signals(6).XData = [0 5 10 15 20 25 30 35 40]
      | sbobj.Groups.Signals(6).YData = [0 0 1 1 1 1 1 1 1]
      | sbobj.Groups.Signals(7).Name = 'Sel_cas'
      | sbobj.Groups.Signals(7).XData = [0 5 10 15 20 25 30 35 40]
      | sbobj.Groups.Signals(7).YData = [1 1 2 3 1 2 3 1 2]
      | sbobj.Groups.Signals(8).Name = 'Fan_Sp_Sel'
      | sbobj.Groups.Signals(8).XData = [0 5 10 15 20 25 30 35 40]
      | sbobj.Groups.Signals(8).YData = [2 2 1 2 3 1 2 3 3]
      | sbobj.Groups.Signals(9).Name = 'Ac_tem_Con'
      | sbobj.Groups.Signals(9).XData = [0 5 10 15 20 25 30 35 40]
      | sbobj.Groups.Signals(9).YData = [25 25 32 25 28 30 20 18 16]
      | sbobj.Groups.Signals(10).Name = 'He_tem_Con'
      | sbobj.Groups.Signals(10).XData = [0 5 10 15 20 25 30 35 40]
      | sbobj.Groups.Signals(10).YData = [12 12 26 35 34 32 35 31 32]
      | sbobj.Groups.Signals(11).Name = 'AIr_Ven'
      | sbobj.Groups.Signals(11).XData = [0 5 10 15 20 25 30 35 40]
      | sbobj.Groups.Signals(11).YData = [50 50 100 50 0 100 0 50 100]
      | sbobj.Groups.TimeRange = [0 40]
  Fr_Do_Cond : Outport  Tag=STV Outport
  Fl_Do_Cond : Outport  Tag=STV Outport  Port=2
  Bl_Do_Cond : Outport  Tag=STV Outport  Port=3
  Br_Do_Cond : Outport  Tag=STV Outport  Port=4
  Fan_Cond : Outport  Tag=STV Outport  Port=5
  Ign_Cond : Outport  Tag=STV Outport  Port=6
  Sel_cas : Outport  Tag=STV Outport  Port=7
  Fan_Sp_Sel : Outport  Tag=STV Outport  Port=8
  Ac_tem_Con : Outport  Tag=STV Outport  Port=9
  He_tem_Con : Outport  Tag=STV Outport  Port=10
  AIr_Ven : Outport  Tag=STV Outport  Port=11
  wires:
  FromWs/1 -> Demux/1
  Demux/1 -> Fr_Do_Cond/1
  Demux/2 -> Fl_Do_Cond/1
  Demux/3 -> Bl_Do_Cond/1
  Demux/4 -> Br_Do_Cond/1
  Demux/5 -> Fan_Cond/1
  Demux/6 -> Ign_Cond/1
  Demux/7 -> Sel_cas/1
  Demux/8 -> Fan_Sp_Sel/1
  Demux/9 -> Ac_tem_Con/1
  Demux/10 -> He_tem_Con/1
  Demux/11 -> AIr_Ven/1

== system Project/IN_Ports/Sunroof_and_InteriorLights_InPorts/Signal Builder2 ==
  Demux : Demux  Tag=STV Demux
      settings: DisplayOption=none
  FromWs : FromWorkspace  Tag=STV FromWs  VariableName=tuvar
      SigBuilderData=|
      | common.afterFinalStr = 'Extrapolate'
      | common.sampleTime = 0
      | dataSet.timeRange = [0 10]
      | dataSet.name = 'Group 1'
      | sbobj.Groups.Name = 'Group 1'
      | sbobj.Groups.Signals(1).Name = 'Fron_Read_Light'
      | sbobj.Groups.Signals(1).XData = [0 0.5 0.5 1 1 1.5 1.5 2 2 2.5 2.5 3 3 3.5 3.5 4 4 4.5 4.5 5 5 5.5 5.5 6 6 6.5 6.5 7 7 7.5 7.5 8 8 8.5 8.5 9 9 9.5 9.5 10]
      | sbobj.Groups.Signals(1).YData = [2 2 0 0 2 2 0 0 2 2 0 0 2 2 0 0 2 2 0 0 2 2 0 0 2 2 0 0 2 2 0 0 2 2 0 0 2 2 0 0]
      | sbobj.Groups.Signals(2).Name = 'Rear_Read_Light'
      | sbobj.Groups.Signals(2).XData = [0 0.5 0.5 1 1 1.5 1.5 2 2 2.5 2.5 3 3 3.5 3.5 4 4 4.5 4.5 5 5 5.5 5.5 6 6 6.5 6.5 7 7 7.5 7.5 8 8 8.5 8.5 9 9 9.5 9.5 10]
      | sbobj.Groups.Signals(2).YData = [2 2 0 0 2 2 0 0 2 2 0 0 2 2 0 0 2 2 0 0 2 2 0 0 2 2 0 0 2 2 0 0 2 2 0 0 2 2 0 0]
      | sbobj.Groups.Signals(3).Name = 'Dome_L'
      | sbobj.Groups.Signals(3).XData = [0 0.5 0.5 1 1 1.5 1.5 2 2 2.5 2.5 3 3 3.5 3.5 4 4 4.5 4.5 5 5 5.5 5.5 6 6 6.5 6.5 7 7 7.5 7.5 8 8 8.5 8.5 9 9 9.5 9.5 10]
      | sbobj.Groups.Signals(3).YData = [2 2 0 0 2 2 0 0 2 2 0 0 2 2 0 0 2 2 0 0 2 2 0 0 2 2 0 0 2 2 0 0 2 2 0 0 2 2 0 0]
      | sbobj.Groups.Signals(4).Name = 'Inst_Light'
      | sbobj.Groups.Signals(4).XData = [0 1 2 3 4 5 6 7 8 9 10]
      | sbobj.Groups.Signals(4).YData = [0 0 1 2 0 2 1 0 1 2 0]
  Fron_Read_Light : Outport  Tag=STV Outport
  Rear_Read_Light : Outport  Tag=STV Outport  Port=2
  Dome_L : Outport  Tag=STV Outport  Port=3
  Inst_Light : Outport  Tag=STV Outport  Port=4
  wires:
  FromWs/1 -> Demux/1
  Demux/1 -> Fron_Read_Light/1
  Demux/2 -> Rear_Read_Light/1
  Demux/3 -> Dome_L/1
  Demux/4 -> Inst_Light/1

== system Project/IN_Ports/Sunroof_and_InteriorLights_InPorts/Signal Builder3 ==
  Demux : Demux  Tag=STV Demux  Outputs=2
      settings: DisplayOption=none
  FromWs : FromWorkspace  Tag=STV FromWs  VariableName=tuvar
      SigBuilderData=|
      | common.afterFinalStr = 'Extrapolate'
      | common.sampleTime = 0
      | dataSet.timeRange = [0 10]
      | dataSet.name = 'Group 1'
      | sbobj.Groups.Name = 'Group 1'
      | sbobj.Groups.Signals(1).Name = 'In_Su_Roof'
      | sbobj.Groups.Signals(1).XData = [0 1 2 3 4 5 6 7 8 9 10]
      | sbobj.Groups.Signals(1).YData = [0 1 2 3 2 1 0 3 0 1 2]
      | sbobj.Groups.Signals(2).Name = 'I_Sensor'
      | sbobj.Groups.Signals(2).XData = [0 1 2 3 4 5 6 7 8 9 10]
      | sbobj.Groups.Signals(2).YData = [0 1 1 0 0 0 0 1 1 0 1]
  In_Su_Roof : Outport  Tag=STV Outport
  I_Sensor : Outport  Tag=STV Outport  Port=2
  wires:
  FromWs/1 -> Demux/1
  Demux/1 -> In_Su_Roof/1
  Demux/2 -> I_Sensor/1

== system Project/IN_Ports/Wiper_and_Power_InPorts/Signal Builder ==
  Demux : Demux  Tag=STV Demux  Outputs=1
      settings: DisplayOption=none
  FromWs : FromWorkspace  Tag=STV FromWs  VariableName=tuvar
      SigBuilderData=|
      | common.afterFinalStr = 'Extrapolate'
      | common.sampleTime = 0
      | dataSet.timeRange = [0 10]
      | dataSet.name = 'Group 1'
      | sbobj.Groups.Name = 'Group 1'
      | sbobj.Groups.Signals.Name = 'Engine_Input'
      | sbobj.Groups.Signals.XData = [0 1 2 3 4 5 6 7 8 9 10 11 12 13 14 15 16 17 18 19 20 21 22 23 24 25]
      | sbobj.Groups.Signals.YData = [0 1 1 0 1 1 0 0 0 1 1 1 0 0 1 0 0 1 0 1 0 0 0 1 1 0]
      | sbobj.Groups.TimeRange = [0 25]
  Engine_Input : Outport  Tag=STV Outport
  wires:
  FromWs/1 -> Demux/1
  Demux/1 -> Engine_Input/1

== system Project/IN_Ports/Wiper_and_Power_InPorts/Signal Builder1 ==
  Demux : Demux  Tag=STV Demux  Outputs=1
      settings: DisplayOption=none
  FromWs : FromWorkspace  Tag=STV FromWs  VariableName=tuvar
      SigBuilderData=|
      | common.afterFinalStr = 'Extrapolate'
      | common.sampleTime = 0
      | dataSet.timeRange = [0 25]
      | dataSet.name = 'Group 1'
      | sbobj.Groups.Name = 'Group 1'
      | sbobj.Groups.Signals.Name = 'In_Value_Wiper'
      | sbobj.Groups.Signals.XData = [0 1 2 3 4 5 6 7 8 9 10 11 12 13 14 15 16 17 18 19 20 21 22 23 24 25]
      | sbobj.Groups.Signals.YData = [1 4 3 4 5 3 1 2 1 4 1 2 5 3 2 3 5 1 4 3 5 1 2 4 3 5]
      | sbobj.Groups.TimeRange = [0 25]
  In_Value_Wiper : Outport  Tag=STV Outport
  wires:
  FromWs/1 -> Demux/1
  Demux/1 -> In_Value_Wiper/1

== system Project/BCM_Car/Alarm_Subsystem/Engine_off_& _Door_close/ SolidOff ==
  Action Port : ActionPort  ActionPortLabel=case [ 0 ]:
  Constant : Constant  Value=0
  Outport : Outport
  wires:
  Constant/1 -> Outport/1

== system Project/BCM_Car/Alarm_Subsystem/Engine_off_& _Door_close/Doors_Locked ==
  Input1 : Inport
  Enable : EnablePort
  Out1 : Outport
  wires:
  Input1/1 -> Out1/1

== system Project/BCM_Car/Alarm_Subsystem/Engine_off_& _Door_close/Doors_Unlocked ==
  Input1 : Inport
  Enable : EnablePort
  Out1 : Outport
  wires:
  Input1/1 -> Out1/1

== system Project/BCM_Car/Alarm_Subsystem/Engine_off_& _Door_close/FasflasH ==
  Action Port : ActionPort  ActionPortLabel=case [ 2 ]:
  Saturation : Saturate  UpperLimit=1  LowerLimit=0
  Signal Generator : SignalGenerator
  Output : Outport
  wires:
  Saturation/1 -> Output/1
  Signal Generator/1 -> Saturation/1

== system Project/BCM_Car/Alarm_Subsystem/Engine_off_& _Door_close/Fast_flash ==
  Action Port : ActionPort  ActionPortLabel=case [ 1 ]:
  Saturation : Saturate  UpperLimit=1  LowerLimit=0
  Signal Generator : SignalGenerator  WaveForm=square
  Output : Outport
  wires:
  Saturation/1 -> Output/1
  Signal Generator/1 -> Saturation/1

== system Project/BCM_Car/Alarm_Subsystem/Engine_off_& _Door_close/Out_Led ==
  Outport : Inport
  Input : Inport  Port=2
  Input1 : Inport  Port=3
  Input2 : Inport  Port=4
  Input3 : Inport  Port=5
  Input4 : Inport  Port=6
  Enable : EnablePort
  Led_checking : Logic  Operator=OR  Inputs=6  IconShape=distinctive  AllPortsSameDT=off  OutDataTypeStr=boolean
  Out1 : Outport
  wires:
  Outport/1 -> Led_checking/1
  Input/1 -> Led_checking/2
  Input1/1 -> Led_checking/3
  Input2/1 -> Led_checking/4
  Input3/1 -> Led_checking/5
  Input4/1 -> Led_checking/6
  Led_checking/1 -> Out1/1

== system Project/BCM_Car/Alarm_Subsystem/Engine_off_& _Door_close/SinglePress _With delay ==
  Action Port : ActionPort  ActionPortLabel=case [ 1 ]:
  Constant1 : Constant
  Delay : Delay  DelayLength=90
  Enabled Subsystem : Subsystem  TreatAsAtomicUnit=on
  Saturation : Saturate  UpperLimit=1  LowerLimit=0
  Signal Generator : SignalGenerator  WaveForm=square  Frequency=0.5
  Step : Step  Time=30  Before=1  After=0  SampleTime=0
  Output : Outport
  wires:
  Enabled Subsystem/1(Out1) -> Output/1
  Delay/1 -> Enabled Subsystem/2(In2)
  Saturation/1 -> Delay/1
  Constant1/1 -> Enabled Subsystem/Enable
  Signal Generator/1 -> Saturation/1
  Step/1 -> Enabled Subsystem/1(In1)

== system Project/BCM_Car/Alarm_Subsystem/Engine_off_& _Door_close/Slow_Flash ==
  Action Port : ActionPort  ActionPortLabel=case [ 2 ]:
  Saturation : Saturate  UpperLimit=1  LowerLimit=0
  Signal Generator : SignalGenerator  WaveForm=square  Frequency=0.5
  Output : Outport
  wires:
  Saturation/1 -> Output/1
  Signal Generator/1 -> Saturation/1

== system Project/BCM_Car/Alarm_Subsystem/Engine_off_& _Door_close/Solid_Off ==
  Action Port : ActionPort  ActionPortLabel=case [ 0 ]:
  Constant : Constant  Value=0
  Output : Outport
  wires:
  Constant/1 -> Output/1

== system Project/BCM_Car/Cruise_Control/If Action Subsystem1/Signal Builder ==
  Demux : Demux  Tag=STV Demux  Outputs=2
      settings: DisplayOption=none
  FromWs : FromWorkspace  Tag=STV FromWs  VariableName=tuvar
      SigBuilderData=|
      | common.afterFinalStr = 'Extrapolate'
      | common.sampleTime = 0
      | dataSet.timeRange = [0 10]
      | dataSet.name = 'Group 1'
      | sbobj.Groups.Name = 'Group 1'
      | sbobj.Groups.Signals(1).Name = 'Plus_Or_Resume'
      | sbobj.Groups.Signals(1).XData = [0 5 5 10 15 20 20 25 30 30 35 35 40 45 50 55 60 65 70 75 80 85 90 95 100]
      | sbobj.Groups.Signals(1).YData = [0 0 1 1 1 1 0 0 0 1 1 0 0 0 0 0 0 0 0 0 0 0 0 0 0]
      | sbobj.Groups.Signals(2).Name = 'Set_Or_Minus'
      | sbobj.Groups.Signals(2).XData = [0 5 10 15 20 20 25 30 30 35 35 40 45 50 55 60 65 70 75 80 85 90 95 100]
      | sbobj.Groups.Signals(2).YData = [0 0 0 0 0 1 1 0 1 1 0 0 0 0 0 0 0 0 0 0 0 0 0 0]
      | sbobj.Groups.TimeRange = [0 100]
  Plus_Or_Resume : Outport  Tag=STV Outport
  Set_Or_Minus : Outport  Tag=STV Outport  Port=2
  wires:
  FromWs/1 -> Demux/1
  Demux/1 -> Plus_Or_Resume/1
  Demux/2 -> Set_Or_Minus/1

== system Project/BCM_Car/Power_Outlet/Power_Outlet_Subsystem/Charging_Subsystem ==
  note: If device starts charging, status is '1'
      | else status is '0'
  In1 : Inport
  Off_Constant_Display : Constant  Value=0
  On_Constant_Display : Constant
  Switch : Switch  Criteria=u2 > Threshold
  tag scope: O_Charging_Status=global
  wires:
  In1/1 -> Switch/2
  On_Constant_Display/1 -> Switch/1
  Off_Constant_Display/1 -> Switch/3
  Switch/1 -> [O_Charging_Status]

== system Project/BCM_Car/do_lock_subsystem/Door_lo_subsystem/Auto_lo_Mode ==
  Action Port : ActionPort  ActionPortLabel=case [ 1 ]:
  lock 3 : Constant
  lock1 : Constant
  lock2 : Constant
  lock4 : Constant
  Out1 : Outport
  Out2 : Outport  Port=2
  Out3 : Outport  Port=3
  Out4 : Outport  Port=4
  wires:
  lock 3/1 -> Out3/1
  lock2/1 -> Out2/1
  lock4/1 -> Out4/1
  lock1/1 -> Out1/1

== system Project/BCM_Car/do_lock_subsystem/Door_lo_subsystem/De_lo_mode ==
  Action Port : ActionPort  ActionPortLabel=case [ 4 ]:
  Enabled Subsystem : Subsystem  TreatAsAtomicUnit=on
  delay : Step  SampleTime=0
  Out1 : Outport
  Output : Outport  Port=2
  Output1 : Outport  Port=3
  Output2 : Outport  Port=4
  wires:
  Enabled Subsystem/1(Out1) -> Out1/1
  delay/1 -> Enabled Subsystem/Enable
  Enabled Subsystem/2(Output) -> Output/1
  Enabled Subsystem/3(Output1) -> Output1/1
  Enabled Subsystem/4(Output2) -> Output2/1

== system Project/BCM_Car/do_lock_subsystem/Door_lo_subsystem/Loc_o_p_mode ==
  Action Port : ActionPort  ActionPortLabel=case [ 2 ]:
  lock 3 : Constant
  lock1 : Constant  Value=0
  lock2 : Constant
  lock4 : Constant
  Out1 : Outport
  Out2 : Outport  Port=2
  Out3 : Outport  Port=3
  Out4 : Outport  Port=4
  wires:
  lock2/1 -> Out2/1
  lock4/1 -> Out4/1
  lock 3/1 -> Out3/1
  lock1/1 -> Out1/1

== system Project/BCM_Car/do_lock_subsystem/Door_lo_subsystem/Rem_Lo_mode ==
  Action Port : ActionPort  ActionPortLabel=case [ 3 ]:
  R_S_Lo_subsystem : Subsystem  TreatAsAtomicUnit=on
  Signal Builder : Subsystem  Tag=STV Subsys  LoadFcn=sigbuilder_block('load');  StartFcn=sigbuilder_block('start');  StopFcn=sigbuilder_block('stop');  ClipboardFcn=sigbuilder_block('clipboard');  mask(Sigbuilder block){tuvar=[0:10]}
      mask help: Simulink:masks:SigbuilderBlock_MD
      mask init:
      | if ~strcmp(get_param(bdroot(gcbh),'SimulationStatus'),'stopped') tuvar = sigbuilder_block('maskInit'); end
      settings: CopyFcn=sigbuilder_block('copy');  DeleteFcn=sigbuilder_block('delete');  ModelCloseFcn=sigbuilder_block('modelClose');  PreSaveFcn=sigbuilder_block('preSave');  PauseFcn=sigbuilder_block('pause');  ContinueFcn=sigbuilder_block('continue');  NameChangeFcn=sigbuilder_block('namechange');  OpenFcn=sigbuilder_block('open',[646.5 174 550.5 399.75 ]);  CloseFcn=sigbuilder_block('close');
      mask Display: plot(0, 0, 100, 100,[2, 2, 32, 32, 2], [68, 8, 8, 68, 68],[32, 2], [38, 38], [32, 19, 2],[53, 60, 44], [32, 17, 17, 2],[16, 16, 31, 31]);txt = getActiveGroup(gcbh);text(2, 100, txt,'verticalAlignment', 'top');
  Outport : Outport
  Output : Outport  Port=2
  Output1 : Outport  Port=3
  Output2 : Outport  Port=4
  wires:
  Signal Builder/1(Sw_Enable) -> R_S_Lo_subsystem/Enable
  R_S_Lo_subsystem/1(Outport) -> Outport/1
  R_S_Lo_subsystem/2(Output) -> Output/1
  R_S_Lo_subsystem/3(Output1) -> Output1/1
  R_S_Lo_subsystem/4(Output2) -> Output2/1

== system Project/BCM_Car/do_lock_subsystem/Door_lo_subsystem/Signal Builder ==
  Demux : Demux  Tag=STV Demux  Outputs=1
      settings: DisplayOption=none
  FromWs : FromWorkspace  Tag=STV FromWs  VariableName=tuvar
      SigBuilderData=|
      | common.afterFinalStr = 'Extrapolate'
      | common.sampleTime = 0
      | dataSet.timeRange = [0 10]
      | dataSet.name = 'Group 1'
      | sbobj.Groups.Name = 'Group 1'
      | sbobj.Groups.Signals.Name = 'Loc_select1'
      | sbobj.Groups.Signals.XData = [0 5 10 15 20 25 30 35 40]
      | sbobj.Groups.Signals.YData = [1 1 2 3 4 1 2 3 4]
  Loc_select1 : Outport  Tag=STV Outport
  wires:
  FromWs/1 -> Demux/1
  Demux/1 -> Loc_select1/1

== system Project/BCM_Car/hvac_subsysytem/ac_he_fan_subsystem/Switch Case Action Subsystem1 ==
  In1 : Inport
  In2 : Inport  Port=2
  In3 : Inport  Port=3
  In4 : Inport  Port=4
  Action Port : ActionPort  ActionPortLabel=case [ 1 ]:
  Out1 : Outport
  Output : Outport  Port=2
  Output1 : Outport  Port=3
  Output2 : Outport  Port=4
  wires:
  In1/1 -> Out1/1
  In2/1 -> Output/1
  In3/1 -> Output1/1
  In4/1 -> Output2/1

== system Project/BCM_Car/hvac_subsysytem/ac_he_fan_subsystem/Switch Case Action Subsystem2 ==
  In1 : Inport
  In2 : Inport  Port=2
  In4 : Inport  Port=3
  In3 : Inport  Port=4
  Action Port : ActionPort  ActionPortLabel=case [ 2 ]:
  Out1 : Outport
  Output : Outport  Port=2
  Output1 : Outport  Port=3
  Output2 : Outport  Port=4
  wires:
  In1/1 -> Out1/1
  In2/1 -> Output/1
  In3/1 -> Output1/1
  In4/1 -> Output2/1

== system Project/BCM_Car/hvac_subsysytem/ac_he_fan_subsystem/Switch Case Action Subsystem3 ==
  In1 : Inport
  In2 : Inport  Port=2
  In3 : Inport  Port=3
  In4 : Inport  Port=4
  Action Port : ActionPort  ActionPortLabel=case [ 3 ]:
  Out1 : Outport
  Output : Outport  Port=2
  Output1 : Outport  Port=3
  Output2 : Outport  Port=4
  wires:
  In1/1 -> Out1/1
  In2/1 -> Output/1
  In3/1 -> Output1/1
  In4/1 -> Output2/1

== system Project/BCM_Car/hvac_subsysytem/ac_he_fan_subsystem/Switch Case Action Subsystem4 ==
  Action Port : ActionPort  ActionPortLabel=case [ 1 ]:
  Constant : Constant
  Out1 : Outport
  wires:
  Constant/1 -> Out1/1

== system Project/BCM_Car/hvac_subsysytem/ac_he_fan_subsystem/Switch Case Action Subsystem5 ==
  Action Port : ActionPort  ActionPortLabel=case [ 2 ]:
  Constant : Constant
  Out1 : Outport
  wires:
  Constant/1 -> Out1/1

== system Project/BCM_Car/hvac_subsysytem/ac_he_fan_subsystem/Switch Case Action Subsystem6 ==
  Action Port : ActionPort  ActionPortLabel=case [ 3 ]:
  Constant : Constant
  Out1 : Outport
  wires:
  Constant/1 -> Out1/1

== system Project/BCM_Car/Alarm_Subsystem/Engine_off_& _Door_close/SinglePress _With delay/Enabled Subsystem ==
  In1 : Inport
  In2 : Inport  Port=2
  Enable : EnablePort
  OR : Logic  Operator=OR  IconShape=distinctive  AllPortsSameDT=off  OutDataTypeStr=boolean
  Out1 : Outport
  wires:
  In1/1 -> OR/1
  In2/1 -> OR/2
  OR/1 -> Out1/1

== system Project/BCM_Car/do_lock_subsystem/Door_lo_subsystem/De_lo_mode/Enabled Subsystem ==
  Enable : EnablePort
  Constant{,1..3} (4 alike) : Constant
  Out1 : Outport
  Output : Outport  Port=2
  Output1 : Outport  Port=3
  Output2 : Outport  Port=4
  wires:
  Constant/1 -> Out1/1
  Constant1/1 -> Output/1
  Constant2/1 -> Output1/1
  Constant3/1 -> Output2/1

== system Project/BCM_Car/do_lock_subsystem/Door_lo_subsystem/Rem_Lo_mode/R_S_Lo_subsystem ==
  Enable : EnablePort
  lock{1..4} (4 alike) : Constant
  Outport : Outport
  Output : Outport  Port=2
  Output1 : Outport  Port=3
  Output2 : Outport  Port=4
  wires:
  lock2/1 -> Output/1
  lock1/1 -> Outport/1
  lock4/1 -> Output2/1
  lock3/1 -> Output1/1

== system Project/BCM_Car/do_lock_subsystem/Door_lo_subsystem/Rem_Lo_mode/Signal Builder ==
  Demux : Demux  Tag=STV Demux  Outputs=1
      settings: DisplayOption=none
  FromWs : FromWorkspace  Tag=STV FromWs  VariableName=tuvar
      SigBuilderData=|
      | common.afterFinalStr = 'Extrapolate'
      | common.sampleTime = 0
      | dataSet.timeRange = [0 100]
      | dataSet.name = 'Group 1'
      | sbobj.Groups.Name = 'Group 1'
      | sbobj.Groups.Signals.Name = 'Sw_Enable'
      | sbobj.Groups.Signals.XData = [0 5 10 15 20 25 30 35 40 45 50 55 60 65 70 75 80 85 90 95 100]
      | sbobj.Groups.Signals.YData = [0 0 0 1 0 0 0 0 1 0 0 0 1 0 0 0 1 0 0 0 1]
      | sbobj.Groups.TimeRange = [0 100]
  Sw_Enable : Outport  Tag=STV Outport
  wires:
  FromWs/1 -> Demux/1
  Demux/1 -> Sw_Enable/1

== stateflow chart Project/BCM_Car/Cruise_Control/If Action Subsystem1/Chart ==
  state main
    during:
    if inc==1
    data=data+1;
    end
    if dec==1
    data=data-1;
    end
  (default) -> main
  data: dec input; inc input; data output =0

== matlab function Project/BCM_Car/Interior_Light/Function_Light ==
  data: u input; y output; u1 input; y1 output; u2 input; y2 output; u3 input; y3 output
function [y,y1,y2,y3] = fcn(u,u1,u2,u3)

y3 = u3;
y2 = u2;
y1 = u1;
y = u;

== matlab function Project/BCM_Car/Sunroof/Function_Sun ==
  data: u input; y output; v input
function y = fcn(u,v)
if u == 1
    for i = 1:5
        y = u * i;
    end
elseif u == 2
    for i = 1:5
        y = u * i;
    end
elseif u == 3
    for i = 1:5
        y = u * i;
    end
else
    y = u;
end
if v == 1 && u ~= 0
   y = 15;
end

== stateflow chart Project/BCM_Car/Hatch_Subsystem/H_B_condition ==
  state Hatch
    entry:
    if hatchButton==1
    y=1;
    end
    if BonnetButton==1
    x=1;
    end
  state Hatch_off
    entry:
    if hatchButton==0
    y=0;
    end
    if BonnetButton==0
    x=0;
    end
  (default) -> Hatch
  Hatch -> Hatch_off : [BonnetButton==0||hatchButton==0]
  Hatch_off -> Hatch : [BonnetButton==1||hatchButton==1]
  data: BonnetButton input; hatchButton input; y output; x output
